simulink model "Tricopter_Controlled"  (R2012b)
settings: Solver=ode3  StartTime=0.0  StopTime=inf  FixedStep=T_sim  MaxStep=0.01  RelTol=1e-5
values from neighbouring files (symbols this model uses):
  A_l_max_x = sqrt( (Max_Thrust*3/m)^2  -  g^2  )    [Run3Copter.m]
  A_x = 0.015    [SetupComplete.m]
  A_y = A_x    (= 0.015)    [SetupComplete.m]
  A_z = 0.16    [SetupComplete.m]
  A_z_max = Max_Thrust*3/m    [Run3Copter.m]
  Alt_0 = input(' Give the initial altitude (m): ')    [Run3Copter.m]
  C_x = 1.2    [SetupComplete.m]
  C_y = C_x    (= 1.2)    [SetupComplete.m]
  C_z = 2.2    [SetupComplete.m]
  CG_0 = [0,0,0.02]'    [SetupComplete.m]
  epsilon = 0.01    [Run3Copter.m]
  eta_1 = deg2rad(-2)    [Run3Copter.m]
  eta_23 = 0    [Run3Copter.m]
  g = 9.81    [SetupComplete.m]
  h_M = 0.064    [SetupComplete.m]
  I_BAC_0 = [ Ix,0,Ixz;0,Iy,0;Ixz,0,Iz]    [SetupComplete.m]
  Initial_Omegas = Omega_hover    [Run3Copter.m]
  Initial_Torques = Torque_hover    [Run3Copter.m]
  Ix = 0.0552    [SetupComplete.m]
  Iy = 0.0552    [SetupComplete.m]
  Iz = 0.11    [SetupComplete.m]
  l = 0.345    [SetupComplete.m]
  l_arm = 0.264    [SetupComplete.m]
  latitude = 52.0733    [Run3Copter.m]
  longitude = 0.6278    [Run3Copter.m]
  m = 3.51    [SetupComplete.m]
  m_0 = 2.61    [SetupComplete.m]
  m_M = 0.300    (= 0.3)    [SetupComplete.m]
  rho = 1.15    [SetupComplete.m]
  Rotation_sign = [ 1,-1,-1]    [SetupComplete.m]
  T_sim = 0.01    [Run3Copter.m]
  throtle_1 = throtle_23/cos(eta_1)    [Run3Copter.m]
  throtle_23 = 0.745    [Run3Copter.m]
  v_i0 = sqrt( 1/3*m*g/(2*rho*pi*R^2)  )    [SetupComplete.m]
undefined symbols (not defined in the file or in its folder): DOWN_0, Earth, EAST_0, Newton, NORTH_0, P_0, Q_0, R_0, Raphson, U_0, V_0, W_0, WGS84
libraries: Adaptive_FaultTolerantControl x24, simulink_extras x11, XXCopter_C x7, XXCopter x5, aerolibfltsims x3, XXCopter_Control x2, qcatlib x1, aerolibconvert2 x1, aerolibtransform2 x1, aerolibanimutils x1, aerolibobsolete x1, simulink x1
(part 1 of 3)
settings Model: ExtModeTrigDuration=5000  Creator=DavidTorres  LastModifiedBy=david.torres
settings SolverCC: SolverResetMethod=Robust  PositivePriorityOrder=on
settings DataIOCC: ExternalInput=getinputstruct(op_trim1)  InitialState=getstatestruct(op_trim1)  SignalLoggingSaveFormat=ModelDataLogs  Refine=10
settings OptimizationCC: InlineParams=on  OptimizeModelRefInitCode=on  LifeSpan=1  SimCompilerOptimization=On
settings DebuggingCC: FcnCallInpInsideContextMsg=UseLocalSettings
settings HardwareCC: ProdIntDivRoundTo=Zero  ProdEndianess=LittleEndian  ProdHWDeviceType=Generic->32-bit x86 compatible
settings RTWCC: SystemTargetFile=ert.tlc  GenCodeOnly=on  TemplateMakefile=RTW.MSVCBuild  Description=Create Visual C/C++ Solution File for the Embedded Coder  ProcessScript=ert_make_rtw_hook
settings CodeAppCC: IgnoreCustomStorageClasses=off
settings ERTTargetCC: CodeReplacementLibrary=C89/C90 (ANSI)  MultiwordLength=2048  GenerateSampleERTMain=on  InlinedParameterPlacement=NonHierarchical  ERTCustomFileTemplate=example_file_process.tlc  ConvertIfToSwitch=off  SuppressUnreachableDefaultCases=off

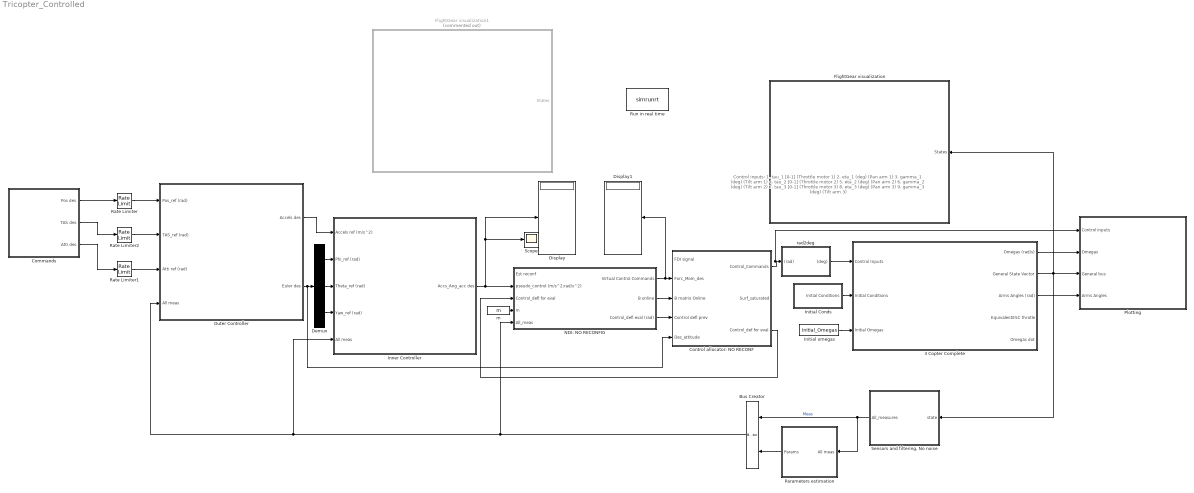
== system Tricopter_Controlled ==
  note: Control inputs:
      | 1. tau_1 [0-1] (Throttle motor 1)
      | 2. eta_1 (deg)  (Pan arm 1)
      | 3. gamma_1 (deg)  (Tilt arm 1)
      |
      | 4. tau_2 [0-1] (Throttle motor 2)
      | 5. eta_2 (deg)  (Pan arm 2)
      | 6. gamma_2 (deg)  (Tilt arm 2)
      |
      | 7. tau_3 [0-1] (Throttle motor 3)
      | 8. eta_3 (deg)  (Pan arm  3)
      | 9. gamma_3 (deg)  (Tilt arm 3)
  3 Copter Complete : Subsystem
      mask Display:
      | image(imread('conv.jpg'))
      | port_label('input', 1, 'Control_in(deg)')
      | port_label('input', 2, 'Ini_condi')
      | port_label('input', 3, 'Ini_Omegas')
      | port_label('output', 1, 'Omegas (rad/s)')
      | port_label('output', 2, 'Gen_state_vec')
      | port_label('output', 3, 'Arms_angl(rad)')
      | port_label('output', 4, 'Eq_ESC_Thro')
      | port_label('output', 5, 'Omegas_dot')
  Bus Creator : BusCreator  Inputs=2
  Commands : Subsystem  TreatAsAtomicUnit=on
  Control allocator: NO RECONF : Subsystem  RTWFcnName=abc  RTWFileName=asas  VariantObject=Control Allocator: NO RECONFIG
      settings: MinAlgLoopOccurrences=on  RTWFcnNameOpts=User specified  RTWFileNameOpts=User specified
  Demux : Demux  Outputs=3
  Display : Display
  Display1 : Display
  FlightGear visualization : Subsystem  TreatAsAtomicUnit=on
      mask Display:
      | disp('{\bf\fontsize{20} Flight Gear}', 'texmode','on');
      | image(imread('convFG.jpg'))
      | port_label('input', 1, 'States')
      | % port_label('input', 2, 'States_dot')
      | % port_label('input', 3, 'Controls')
  FlightGear visualization1 : Subsystem  Commented=on  TreatAsAtomicUnit=on
      mask Display:
      | disp('{\bf\fontsize{20} Flight Gear}', 'texmode','on');
      | image(imread('convFG.jpg'))
      | port_label('input', 1, 'States')
      | % port_label('input', 2, 'States_dot')
      | % port_label('input', 3, 'Controls')
  Initial Conds : Subsystem  TreatAsAtomicUnit=on
  Initial omegas : Constant  Value=Initial_Omegas
  Inner Controller : Subsystem  Variant=on  OverrideUsingVariant=PI
  NDI: NO RECONFIG : Subsystem  RTWFcnName=abc  RTWFileName=asas  VariantObject=NDI: NO RECONFIG
      settings: RTWFcnNameOpts=User specified  RTWFileNameOpts=User specified
  Outer Controller : Subsystem  Variant=on  OverrideUsingVariant=Overactuated P Controller
  Parameters estimation : Subsystem  TreatAsAtomicUnit=on
  Plotting : Subsystem
  Rate Limiter : RateLimiter  RisingSlewLimit=5  FallingSlewLimit=-5  SampleTimeMode=inherited
  Rate Limiter1 : RateLimiter  RisingSlewLimit=0.2  FallingSlewLimit=-0.2  SampleTimeMode=inherited
  Rate Limiter2 : RateLimiter  RisingSlewLimit=10  FallingSlewLimit=-10  SampleTimeMode=inherited
  Run in real time : S-Function  FunctionName=simrunrt  Parameters=1  EnableBusSupport=off
  Scope : Scope
      settings: YMin=-2  YMax=8  SaveName=ScopeData3
  Sensors and filtering. No noise : Subsystem  VariantObject=No noise
  m : Constant  Value=m
  rad2deg : Subsystem  TreatAsAtomicUnit=on
  wires:
  Initial omegas/1 -> 3 Copter Complete/3(Initial Omegas)
  Initial Conds/1(Initial Conditions) -> 3 Copter Complete/2(Initial Conditions)
  3 Copter Complete/2(General State Vector) -> Sensors and filtering. No noise/1(state), Plotting/3(General bus), FlightGear visualization/1(States)
  3 Copter Complete/1(Omegas (rad/s)) -> Plotting/2(Omegas)
  Control allocator: NO RECONF/1(Control_Commands) -> Plotting/1(Control inputs), rad2deg/1((rad))
  NDI: NO RECONFIG/1(Virtual Control Commands) -> Display1/1, Control allocator: NO RECONF/2(Forc_Mom_des)
  Control allocator: NO RECONF/3(Control_def for eval) -> NDI: NO RECONFIG/3(Control_defl for eval)
  m/1 -> NDI: NO RECONFIG/4(m)
  NDI: NO RECONFIG/3(Control_defl eval (rad)) -> Control allocator: NO RECONF/4(Control defl prev)
  rad2deg/1((deg)) -> 3 Copter Complete/1(Control Inputs)
  Sensors and filtering. No noise/1(All_measures) -> Parameters estimation/1(All meas), Bus Creator/1  "Meas"
  NDI: NO RECONFIG/2(B online) -> Control allocator: NO RECONF/3(B matrix Online)
  Inner Controller/1(Accs_Ang_acc des) -> Display/1, Scope/1, NDI: NO RECONFIG/2(pseudo_control (m/s^2;rad/s^2))
  Parameters estimation/1(Params) -> Bus Creator/2
  3 Copter Complete/3(Arms Angles (rad)) -> Plotting/4(Arms Angles)
  Bus Creator/1 -> Outer Controller/4(All meas), Inner Controller/5(All meas), NDI: NO RECONFIG/5(All_meas)
  Outer Controller/2(Euler des) -> Control allocator: NO RECONF/5(Des_attitude), Demux/1
  Demux/3 -> Inner Controller/4(Yaw_ref (rad))
  Demux/2 -> Inner Controller/3(Theta_ref (rad))
  Demux/1 -> Inner Controller/2(Phi_ref (rad))
  Outer Controller/1(Accels des) -> Inner Controller/1(Accels ref (m/s^2))
  Commands/1(Pos des) -> Rate Limiter/1
  Rate Limiter/1 -> Outer Controller/1(Pos_ref (rad))
  Commands/3(Atti des) -> Rate Limiter1/1
  Rate Limiter1/1 -> Outer Controller/3(Atti ref (rad))
  Rate Limiter2/1 -> Outer Controller/2(TAS_ref (rad))
  Commands/2(TAS des) -> Rate Limiter2/1

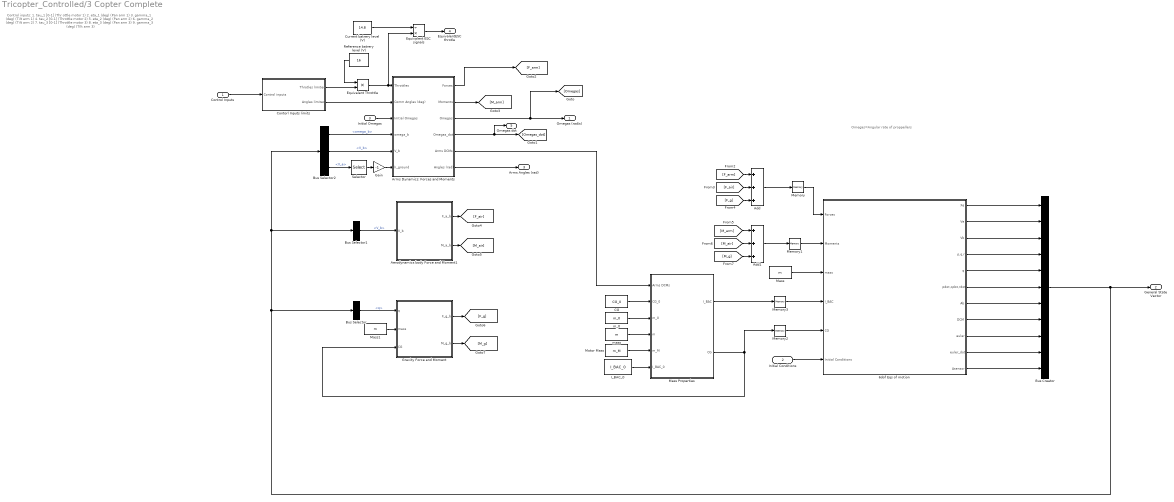
== system Tricopter_Controlled/3 Copter Complete ==
  note: Omegas=Angular rate of proppellers
  note: Control inputs:
      | 1. tau_1 [0-1] (Thr ottle motor 1)
      | 2. eta_1 (deg)  (Pan arm 1)
      | 3. gamma_1 (deg)  (Tilt arm 1)
      |
      | 4. tau_2 [0-1] (Throttle motor 2)
      | 5. eta_2 (deg)  (Pan arm 2)
      | 6. gamma_2 (deg)  (Tilt arm 2)
      |
      | 7. tau_3 [0-1] (Throttle motor 3)
      | 8. eta_3 (deg)  (Pan arm  3)
      | 9. gamma_3 (deg)  (Tilt arm 3)
  Control Inputs : Inport
  Initial Conditions : Inport  Port=2
  Initial Omegas : Inport  Port=3
  6dof Eqs of motion : Subsystem  TreatAsAtomicUnit=on
  Add : Sum  Inputs=+++
  Add1 : Sum  Inputs=+++
  Aerodynamics body Force and Moment1 : MATLAB Function  TreatAsAtomicUnit=on
      settings: PermitHierarchicalResolution=ParametersOnly
  Arms Dynamics: Forces and Moments : Subsystem
  Bus Creator : BusCreator  Inputs=11
  Bus Selector : BusSelector  OutputSignals=q
  Bus Selector1 : BusSelector  OutputSignals=V_b
  Bus Selector2 : BusSelector  OutputSignals=omega_b,V_b,X_e
  CG : Constant  Value=CG_0
  Contorl Inputs limits : Subsystem  TreatAsAtomicUnit=on
  Current batrery level (V) : Constant  Value=14.8
  Equivalent ESC signals : Product  Inputs=/*
  Equivalent Throttle : Product  Inputs=**
  Gain : Gain  Gain=-1
  Gravity Force and Moment : MATLAB Function  TreatAsAtomicUnit=on
      settings: PermitHierarchicalResolution=ParametersOnly
  I_BAC_0 : Constant  Value=I_BAC_0
  Mass : Constant  Value=m
  Mass Properties : Subsystem  TreatAsAtomicUnit=on
  Mass1 : Constant  Value=m
  Memory : Memory  X0=[0,0,0]
  Memory1 : Memory  X0=[0,0,0]
  Memory2 : Memory  X0=CG_0
  Memory3 : Memory  X0=I_BAC_0
  Motor Mass : Constant  Value=m_M
  Reference batrery level (V) : Constant  Value=16
  Selector : Selector  InputPortWidth=3  Indices=3
  m_0 : Constant  Value=m_0
  mass : Constant  Value=m
  Omegas (rad/s) : Outport
  General State Vector : Outport  Port=2
  Arms Angles (rad) : Outport  Port=3
  EquivalentESC throtle : Outport  Port=4
  Omegas dot : Outport  Port=5
  wires:
  Initial Conditions/1 -> 6dof Eqs of motion/6(Initial Conditions)
  6dof Eqs of motion/3(Vb) -> Bus Creator/3
  6dof Eqs of motion/5(q) -> Bus Creator/5
  6dof Eqs of motion/2(Ve) -> Bus Creator/2
  6dof Eqs of motion/6(pdot,qdot,rdot) -> Bus Creator/6
  6dof Eqs of motion/1(Xe) -> Bus Creator/1
  6dof Eqs of motion/7(Ab) -> Bus Creator/7
  6dof Eqs of motion/8(DCM) -> Bus Creator/8
  6dof Eqs of motion/9(euler) -> Bus Creator/9
  6dof Eqs of motion/10(euler_dot) -> Bus Creator/10
  Bus Selector/1 -> Gravity Force and Moment/1(q)  "<q>"
  Mass/1 -> 6dof Eqs of motion/3(mass)
  Mass Properties/1(I_BAC) -> Memory3/1
  Bus Selector1/1 -> Aerodynamics body Force and Moment1/1(V_b)  "<V_b>"
  Bus Selector2/1 -> Arms Dynamics: Forces and Moments/4(omega_b)  "<omega_b>"
  Bus Selector2/2 -> Arms Dynamics: Forces and Moments/5(V_b)  "<V_b>"
  Mass1/1 -> Gravity Force and Moment/2(mass)
  Mass Properties/2(CG) -> Gravity Force and Moment/3(CG), Memory2/1
  Arms Dynamics: Forces and Moments/4(Omegas_dot) -> Omegas dot/1, [Omegas_dot]
  Initial Omegas/1 -> Arms Dynamics: Forces and Moments/3(Initial Omegas)
  Bus Selector2/3 -> Selector/1  "<X_e>"
  Selector/1 -> Gain/1
  Gain/1 -> Arms Dynamics: Forces and Moments/6(h_ground)
  Add/1 -> Memory/1
  Add1/1 -> Memory1/1
  Arms Dynamics: Forces and Moments/1(Forces) -> [F_arm]
  Arms Dynamics: Forces and Moments/2(Moments) -> [M_arm]
  Aerodynamics body Force and Moment1/1(F_a_b) -> [F_air]
  Aerodynamics body Force and Moment1/2(M_a_b) -> [M_air]
  Gravity Force and Moment/1(F_g_b) -> [F_g]
  Gravity Force and Moment/2(M_g_b) -> [M_g]
  [F_arm] -> Add/1
  [F_air] -> Add/2
  [F_g] -> Add/3
  [M_arm] -> Add1/1
  [M_g] -> Add1/3
  [M_air] -> Add1/2
  6dof Eqs of motion/11(Asensor) -> Bus Creator/11
  Contorl Inputs limits/1(Throtles limited) -> Equivalent Throttle/2
  Contorl Inputs limits/2(Angles limited) -> Arms Dynamics: Forces and Moments/2(Comm Angles (deg))
  Arms Dynamics: Forces and Moments/5(Arms DCMs) -> Mass Properties/1(Arms DCMs)
  CG/1 -> Mass Properties/2(CG_0)
  Motor Mass/1 -> Mass Properties/5(m_M)
  I_BAC_0/1 -> Mass Properties/6(I_BAC_0)
  m_0/1 -> Mass Properties/3(m_0)
  mass/1 -> Mass Properties/4(m)
  Arms Dynamics: Forces and Moments/3(Omegas) -> [Omegas], Omegas (rad/s)/1
  Bus Creator/1 -> Bus Selector2/1, Bus Selector1/1, Bus Selector/1, General State Vector/1
  Memory/1 -> 6dof Eqs of motion/1(Forces)
  Memory1/1 -> 6dof Eqs of motion/2(Moments)
  Memory2/1 -> 6dof Eqs of motion/5(CG)
  Memory3/1 -> 6dof Eqs of motion/4(I_BAC)
  Equivalent Throttle/1 -> Equivalent ESC signals/2, Arms Dynamics: Forces and Moments/1(Throttles)
  Reference batrery level (V)/1 -> Equivalent Throttle/1
  Current batrery level (V)/1 -> Equivalent ESC signals/1
  Equivalent ESC signals/1 -> EquivalentESC throtle/1
  6dof Eqs of motion/4(p,q,r) -> Bus Creator/4
  Arms Dynamics: Forces and Moments/6(Angles (rad)) -> Arms Angles (rad)/1
  Control Inputs/1 -> Contorl Inputs limits/1(Control inputs)

== system Tricopter_Controlled/Commands ==
  Ini Position X_e_0 : Constant  Value=[0;0;-Alt_0-10]
  Ini Position X_e_1 : Constant  Value=[0;0;-Alt_0]
  Initial Attitude Euler_0 : Constant  Value=[deg2rad(0);deg2rad(0);deg2rad(90)]  SampleTime=-1
  Initial Attitude Euler_1 : Constant  Value=[deg2rad(0);deg2rad(0);deg2rad(0)]
  Manual Switch : ManualSwitch  CurrentSetting=0
  Manual Switch1 : ManualSwitch
  Manual Switch2 : ManualSwitch  CurrentSetting=0
  Veas des : Constant  Value=0
  Veas des1 : Constant  Value=10
  Pos des : Outport
  TAS des : Outport  Port=2
  Atti des : Outport  Port=3
  wires:
  Manual Switch1/1 -> Pos des/1
  Manual Switch/1 -> Atti des/1
  Initial Attitude Euler_0/1 -> Manual Switch/1
  Initial Attitude Euler_1/1 -> Manual Switch/2
  Ini Position X_e_0/1 -> Manual Switch1/1
  Ini Position X_e_1/1 -> Manual Switch1/2
  Manual Switch2/1 -> TAS des/1
  Veas des1/1 -> Manual Switch2/1
  Veas des/1 -> Manual Switch2/2

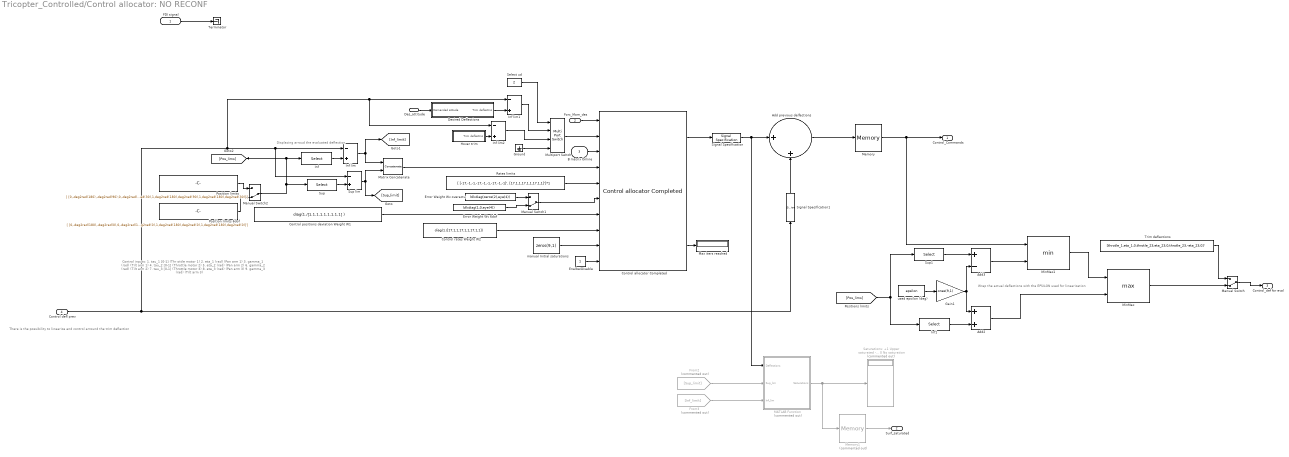
== system Tricopter_Controlled/Control allocator: NO RECONF ==
  note: There is the possibility to linearize and control arround the trim deflection
  note: Wrap the actual deflections with the EPSILON
      |  used for linearization
  note: Displacing arroud the evaluated deflection
  note: Control inputs:
      | 1. tau_1 [0-1] (Thr ottle motor 1)
      | 2. eta_1 (rad)  (Pan arm 1)
      | 3. gamma_1 (rad)  (Tilt arm 1)
      |
      | 4. tau_2 [0-1] (Throttle motor 2)
      | 5. eta_2 (rad)  (Pan arm 2)
      | 6. gamma_2 (rad)  (Tilt arm 2)
      |
      | 7. tau_3 [0-1] (Throttle motor 3)
      | 8. eta_3 (rad)  (Pan arm  3)
      | 9. gamma_3 (rad)  (Tilt arm 3)
  FDI signal : Inport
  Forc_Mom_des : Inport  Port=2
  B matrix Online : Inport  Port=3
  Control defl prev : Inport  Port=4
  Des_attitude : Inport  Port=5
  Add previous delfections : Sum  Inputs=|++
  Add2 : Sum
  Add3 : Sum  Inputs=+-
  "Control allocator Completed " : qcatlib/Control allocator Completed   alg=WLS  CA_type=QP  iter_max=100  gamma=1  k_B=6  m_B=9  T=T_sim  tol=1e-5
  Control positions deviation Weight W1 : Constant  Value=diag(1./[1,1,1,1,1,1,1,1,1] )
  Control rates Weight W2 : Constant  Value=diag(1./[17,1,1,17,1,1,17,1,1])
  Desired Deflections : Subsystem  TreatAsAtomicUnit=on
  Enalbe/Disable : Constant
  Error Weight Wv 6dof : Constant  Value=blkdiag(1,0,eye(4))
  Error Weight Wv overactu : Constant  Value=blkdiag(zeros(2),eye(4))
  From2 : From  Commented=on  GotoTag=Sup_limit
  From3 : From  Commented=on  GotoTag=Inf_limit
  Gain1 : Gain  Gain=ones(9,1)
  Ground : Ground
  Hover trim : Subsystem  TreatAsAtomicUnit=on
  Inf : Selector  NumberOfDimensions=2  InputPortWidth=3  IndexOptions=Index vector (dialog),Index vector (dialog)  Indices=[1:9],1  OutputSizes=1,1
  Inf lim : Sum  Inputs=-+
  Inf lim1 : Sum  Inputs=-+
  Inf lim2 : Sum  Inputs=-+
  Inf1 : Selector  NumberOfDimensions=2  InputPortWidth=3  IndexOptions=Index vector (dialog),Index vector (dialog)  Indices=[1:9],1  OutputSizes=1,1
  MATLAB Function : MATLAB Function  Commented=on  TreatAsAtomicUnit=on
      settings: PermitHierarchicalResolution=ParametersOnly
  Manual Switch : ManualSwitch  CurrentSetting=0
  Manual Switch1 : ManualSwitch  CurrentSetting=0
  Manual Switch2 : ManualSwitch  CurrentSetting=0
  Matrix Concatenate : Concatenate  Mode=Multidimensional array  ConcatenateDimension=2
  Max iters reached : Display
  Memory : Memory  X0=[throtle_1,eta_1,0,throtle_23,eta_23,0,throtle_23,-eta_23,0]'
  Memory1 : Memory  Commented=on  X0=zeros(7,1)
  MinMax : MinMax  Function=max  Inputs=2
  MinMax1 : MinMax  Inputs=2
  Multiport Switch : MultiPortSwitch
  Position limits : Constant  Value=[ [0,-deg2rad(180),-deg2rad(90),0,-deg2rad(180),-deg2rad(30),0,-deg2rad(180),-deg2rad(90)]', [1,deg2rad(180),deg2rad(30),1,deg2rad(180),deg2rad(90),1,deg2rad(180),deg2rad(30)]']
  Position limits 6dof : Constant  Value=[ [0,-deg2rad(180),-deg2rad(0),0,-deg2rad(180),-deg2rad(0),0,-deg2rad(180),-deg2rad(0)]', [1,deg2rad(180),deg2rad(0),1,deg2rad(180),deg2rad(0),1,deg2rad(180),deg2rad(0)]']
  Rates limits : Constant  Value=[ [-17,-1,-1,-17,-1,-1,-17,-1,-1]', [17,1,1,17,1,1,17,1,1]']*1
  Saturations: +1 Upper saturated -1 Lower saturated 0 No saturation : Display  Commented=on
  Select ud : Constant  Value=2
  Signal Specification : SignalSpecification  Dimensions=[9,1]
  Signal Specification1 : SignalSpecification  Dimensions=[9,1]
  Sup : Selector  NumberOfDimensions=2  InputPortWidth=3  IndexOptions=Index vector (dialog),Index vector (dialog)  Indices=[1:9],2  OutputSizes=1,1
  Sup lim : Sum  Inputs=-+
  Sup1 : Selector  NumberOfDimensions=2  InputPortWidth=3  IndexOptions=Index vector (dialog),Index vector (dialog)  Indices=[1:9],2  OutputSizes=1,1
  Terminator : Terminator
  "Trim deflections " : Constant  Value=[throtle_1,eta_1,0,throtle_23,eta_23,0,throtle_23,-eta_23,0]'
  manual Initial saturations : Constant  Value=zeros(9,1)
  used epsilon (deg) : Constant  Value=epsilon
  Control_Commands : Outport
  Surf_saturated : Outport  Port=2
  Control_def for eval : Outport  Port=3
  wires:
  Manual Switch/1 -> Control_def for eval/1
  MinMax1/1 -> MinMax/1
  Add3/1 -> MinMax1/2
  used epsilon (deg)/1 -> Gain1/1
  Inf1/1 -> Add2/2
  Gain1/1 -> Add3/2, Add2/1
  Sup1/1 -> Add3/1
  Add2/1 -> MinMax/2
  Add previous delfections/1 -> Memory/1
  Control positions deviation Weight W1/1 -> "Control allocator Completed "/7
  FDI signal/1 -> Terminator/1
  "Control allocator Completed "/1 -> Signal Specification/1
  Enalbe/Disable/1 -> "Control allocator Completed "/10
  manual Initial saturations/1 -> "Control allocator Completed "/9
  "Control allocator Completed "/3 -> Max iters reached/1
  Sup lim/1 -> [Sup_limit], Matrix Concatenate/2
  Inf lim/1 -> [Inf_limit], Matrix Concatenate/1
  Inf/1 -> Inf lim/2
  Sup/1 -> Sup lim/2
  Control rates Weight W2/1 -> "Control allocator Completed "/8
  Manual Switch1/1 -> "Control allocator Completed "/6
  Rates limits/1 -> "Control allocator Completed "/5
  Manual Switch2/1 -> Inf/1, [Pos_lims], Sup/1
  Memory/1 -> MinMax1/1, Control_Commands/1
  From2/1 -> MATLAB Function/2(Sup_lim)
  From3/1 -> MATLAB Function/3(Inf_lim)
  MATLAB Function/1(Saturations) -> Memory1/1, Saturations: +1 Upper saturated -1 Lower saturated 0 No saturation/1
  Memory1/1 -> Surf_saturated/1
  B matrix Online/1 -> "Control allocator Completed "/3
  Signal Specification/1 -> MATLAB Function/1(Deflections), Add previous delfections/1
  Signal Specification1/1 -> Add previous delfections/2
  Desired Deflections/1(Trim deflectins) -> Inf lim1/2
  [Pos_lims] -> Sup1/1, Inf1/1
  Forc_Mom_des/1 -> "Control allocator Completed "/1
  "Trim deflections "/1 -> Manual Switch/1
  MinMax/1 -> Manual Switch/2
  Matrix Concatenate/1 -> "Control allocator Completed "/4
  Multiport Switch/1 -> "Control allocator Completed "/2
  Error Weight Wv overactu/1 -> Manual Switch1/1
  Des_attitude/1 -> Desired Deflections/1(Demanded atitude)
  Hover trim/1(Trim deflectins) -> Inf lim2/2
  Control defl prev/1 -> Signal Specification1/1, Inf lim2/1, Inf lim1/1, Inf lim/1, Sup lim/1
  Inf lim1/1 -> Multiport Switch/2
  Inf lim2/1 -> Multiport Switch/3
  Ground/1 -> Multiport Switch/4
  Select ud/1 -> Multiport Switch/1
  Position limits 6dof/1 -> Manual Switch2/2
  Position limits/1 -> Manual Switch2/1
  Error Weight Wv 6dof/1 -> Manual Switch1/2

== system Tricopter_Controlled/FlightGear visualization ==
  States : Inport
  Bus Selector : BusSelector  OutputSignals=X_e,euler
  Demux : Demux  Outputs=3
  Flat Earth to LLA : Subsystem
  Mux : Mux  Inputs=6
  Saturation : Saturate  UpperLimit=1e8  LowerLimit=-1e5  OutDataTypeStr=double
  Send2FG : S-Function  FunctionName=sim2fg  Parameters='localhost',5502  EnableBusSupport=off
  cast1 : DataTypeConversion  OutDataTypeStr=double  SaturateOnIntegerOverflow=on
  href : Constant  Value=Alt_0  VectorParams1D=off
  keep pi/pi : Subsystem
  wires:
  States/1 -> Bus Selector/1
  Demux/2 -> Mux/5
  Demux/1 -> Mux/4
  href/1 -> Flat Earth to LLA/2(altitude0)
  Saturation/1 -> Mux/3
  Mux/1 -> cast1/1
  cast1/1 -> Send2FG/1
  keep pi/pi/1(ptp_earth) -> Demux/1
  Demux/3 -> Mux/6
  Flat Earth to LLA/3(altitude h) -> Saturation/1
  Flat Earth to LLA/1(latitude mu) -> Mux/1
  Flat Earth to LLA/2(longitude l) -> Mux/2
  Bus Selector/2 -> keep pi/pi/1(phi theta psi)  "<euler>"
  Bus Selector/1 -> Flat Earth to LLA/1(Xe)  "<X_e>"

== system Tricopter_Controlled/FlightGear visualization1 ==
  States : Inport
  Bus Selector : BusSelector  OutputSignals=X_e,omega_b,euler
  Demux : Demux  Outputs=3
  Flat Earth to LLA : Subsystem
  Generate Run Script (Cranfield Airport) : aerolibfltsims/Generate Run Script  OutputFileName=runfg.bat  FlightGearBaseDirectory=C:\Program Files\FlightGear  GeometryModelName=f16  DestinationPort=5502  OriginAddress=127.0.0.1  OriginPort=5505  LocalAddress=127.0.0.1  AirportId=EGTC  RunwayId=1  InitialAltitude=Alt_0*3.2808399  InitialHeading=0  OffsetDistance=1  OffsetAzimuth=0  GenerateFile=off  Architecture=Win64  dataFlow=Send
  Pack net_fdm Packet for FlightGear : aerolibfltsims/Pack net_fdm Packet for FlightGear  FlightGearVersion=v2.6  ShowPositionAttitudeInputs=on  ShowVelocityAccelerationInputs=off  ShowControlSurfacePositionInputs=off  ShowEngineFuelInputs=off  ShowLandingGearInputs=off  ShowEnvironmentInputs=off  SampleTime=-1
      settings: AttributesFormatString=FG VERSION: %<FlightGearVersion>
  Saturation : Saturate  UpperLimit=1e8  LowerLimit=-1e5
  Send net_fdm Packet to FlightGear : aerolibfltsims/Send net_fdm Packet to FlightGear  DestinationIpAddress=127.0.0.1  DestinationPort=5502  LocalIpPort=-1  varLen=off  SampleTime=-1
  Simulation Pace : aerolibanimutils/Simulation Pace  SimulationPace=1  SleepMode=MATLAB Thread  OutputPaceError=off  SampleTime=4*T_sim
      settings: AttributesFormatString=%<SimulationPace> sec/sec
  cast2 : DataTypeConversion  OutDataTypeStr=single  SaturateOnIntegerOverflow=on
  href : Constant  Value=Alt_0  VectorParams1D=off
  phidot thetadot psidot : Subsystem
  wires:
  Bus Selector/3 -> phidot thetadot psidot/2(phi theta psi)  "<euler>"
  Bus Selector/2 -> phidot thetadot psidot/1(pqr)  "<omega_b>"
  Bus Selector/1 -> Flat Earth to LLA/1(Xe)  "<X_e>"
  States/1 -> Bus Selector/1
  Demux/3 -> Pack net_fdm Packet for FlightGear/6
  Demux/2 -> Pack net_fdm Packet for FlightGear/5
  Demux/1 -> Pack net_fdm Packet for FlightGear/4
  Saturation/1 -> Pack net_fdm Packet for FlightGear/3
  cast2/1 -> Demux/1
  Flat Earth to LLA/2(latitude mu) -> Pack net_fdm Packet for FlightGear/2
  Flat Earth to LLA/1(longitude l) -> Pack net_fdm Packet for FlightGear/1
  Flat Earth to LLA/3(altitude h) -> Saturation/1
  href/1 -> Flat Earth to LLA/2(altitude0)
  phidot thetadot psidot/1(ptp_earth) -> cast2/1
  Pack net_fdm Packet for FlightGear/1 -> Send net_fdm Packet to FlightGear/1

== system Tricopter_Controlled/Initial Conds ==
  Bus Creator : BusCreator
  Ini Position X_e_0 : Constant  Value=[0;0;-Alt_0]
  Initial Attitude Euler_0 : Constant  Value=[deg2rad(0);deg2rad(0);deg2rad(0)]
  Initial Attitude Rate  Euler_dot_0 : Constant  Value=[deg2rad(0);deg2rad(0);deg2rad(0)]
  Initial Velocity V_e_0 : Constant  Value=[0;0;0]
  Initial Conditions : Outport
  wires:
  Ini Position X_e_0/1 -> Bus Creator/1  "X_e_0"
  Initial Velocity V_e_0/1 -> Bus Creator/2  "V_e_0"
  Initial Attitude Euler_0/1 -> Bus Creator/3  "Euler_0"
  Initial Attitude Rate  Euler_dot_0/1 -> Bus Creator/4  "Euler_dot_0"
  Bus Creator/1 -> Initial Conditions/1

== system Tricopter_Controlled/Inner Controller ==
  note: 1) Only subsystems can be added as variant choices at this level
      | 2) Blocks cannot be connected at this level as connectivity is
      | automatically determined at simulation, based on the active variant
  Accels ref (m/s^2) : Inport
  Phi_ref (rad) : Inport  Port=2
  Theta_ref (rad) : Inport  Port=3
  Yaw_ref (rad) : Inport  Port=4
  All meas : Inport  Port=5
  P Controller : Subsystem  VariantObject=P
  PI Controller : Subsystem  VariantObject=PI
  Accs_Ang_acc des : Outport

== system Tricopter_Controlled/NDI: NO RECONFIG ==
  note: Rejection for the
      | angular accelerations
  note: Pseudo control inputs:
      | 1. Desired angular accelerations (rad/s^2)
      | 2. Desired accelerations (m/s^2) in body axes
  Est reconf : Inport
  pseudo_control (m/s^2;rad/s^2) : Inport  Port=2
  Control_defl for eval : Inport  Port=3
  m : Inport  Port=4
  All_meas : Inport  Port=5
  3Copter_4_NDI&CA : Subsystem  AncestorBlock=XXCopter_Control/3Copter_4_NDI&CA  TreatAsAtomicUnit=on
  Bus Selector : BusSelector  OutputSignals=Meas.omega_b meas (rad/s),Meas.q_meas,Meas.V_b_meas,Meas.Alt meas (m)
  Demux : Demux  Outputs=[3,3]
  Derivative1 : Derivative  CoefficientInTFapproximation=500
  Gain : Gain  Gain=[1,0,1]
  Gain1 : Gain  Gain=[1,0,1]'
  Ground : Ground
  Ground1 : Ground
  Inversion : Sum  Inputs=|+-
  Mux : Mux  Inputs=[3,3]
  Mux2 : Mux  Inputs=[3,3]
  Rot eqs_ Get moments : XXCopter_Control/Rot eqs_ Get moments
  Terminator : Terminator
  Transl Eqs_ Get forces : XXCopter_Control/Transl Eqs_ Get forces
  "angles " : Selector  IndexMode=Zero-based  InputPortWidth=9  Indices=[1,2,4,5,7,8]
  epsilon (rad or unitary) : Constant  Value=epsilon
  m1 : InportShadow  Port=4
  Virtual Control Commands : Outport
  B online : Outport  Port=2
  Control_defl eval (rad) : Outport  Port=3
  wires:
  Est reconf/1 -> Terminator/1
  3Copter_4_NDI&CA/3(CA_grad) -> B online/1
  Mux/1 -> Inversion/1
  Mux2/1 -> Inversion/2  "f_x(x)"
  All_meas/1 -> Bus Selector/1
  pseudo_control (m/s^2;rad/s^2)/1 -> Demux/1
  Demux/2 -> Rot eqs_ Get moments/2, Transl Eqs_ Get forces/4
  Demux/1 -> Transl Eqs_ Get forces/1
  Bus Selector/1 -> Transl Eqs_ Get forces/3, Rot eqs_ Get moments/1, 3Copter_4_NDI&CA/6(omega_b)  "<omega_b meas (rad/s)>"
  Bus Selector/3 -> Transl Eqs_ Get forces/2, 3Copter_4_NDI&CA/4(Vb)  "<V_b_meas>"
  3Copter_4_NDI&CA/4(I_BAC) -> Rot eqs_ Get moments/3
  3Copter_4_NDI&CA/5("CG ") -> Transl Eqs_ Get forces/6
  Control_defl for eval/1 -> 3Copter_4_NDI&CA/2(Control Inputs (rad)), Control_defl eval (rad)/1, "angles "/1
  Bus Selector/4 -> 3Copter_4_NDI&CA/3(h)  "<Alt meas (m)>"
  Bus Selector/2 -> 3Copter_4_NDI&CA/5(q)  "<q_meas>"
  m/1 -> 3Copter_4_NDI&CA/11(" m")
  m1/1 -> Transl Eqs_ Get forces/5
  epsilon (rad or unitary)/1 -> 3Copter_4_NDI&CA/1("epsilon (rad or unitary) ")
  Transl Eqs_ Get forces/1 -> Gain1/1
  Rot eqs_ Get moments/1 -> Mux/2
  3Copter_4_NDI&CA/1(Forces) -> Gain/1
  3Copter_4_NDI&CA/2(Moments) -> Mux2/2
  Inversion/1 -> Virtual Control Commands/1
  Ground/1 -> 3Copter_4_NDI&CA/7(Omegas_dot_actual)
  "angles "/1 -> Derivative1/1, 3Copter_4_NDI&CA/8(angles_actual)
  Derivative1/1 -> 3Copter_4_NDI&CA/9(angles_dot_actual)
  Ground1/1 -> 3Copter_4_NDI&CA/10(angles_dot_dot_actual)
  Gain/1 -> Mux2/1
  Gain1/1 -> Mux/1

== system Tricopter_Controlled/Outer Controller ==
  note: 1) Only subsystems can be added as variant choices at this level
      | 2) Blocks cannot be connected at this level as connectivity is
      | automatically determined at simulation, based on the active variant
  Pos_ref (rad) : Inport
  TAS_ref (rad) : Inport  Port=2
  Atti ref (rad) : Inport  Port=3
  All meas : Inport  Port=4
  Overactuated P Controller : Subsystem  VariantObject=Overactuated P Controller
  Underactuated P Controller : Subsystem  VariantObject=Underactuated P Controller
  Accels des : Outport
  Euler des : Outport  Port=2

== system Tricopter_Controlled/Parameters estimation ==
  All meas : Inport
  Bus Selector : BusSelector  OutputSignals=Euler meas (rad)
  DCM1 : Subsystem  TreatAsAtomicUnit=on
  Selector7 : Selector  InputPortWidth=3  Indices=[3 2 1]
  Params : Outport
  wires:
  All meas/1 -> Bus Selector/1
  Bus Selector/1 -> Selector7/1  "<Euler meas (rad)>"
  DCM1/1(DCM) -> Params/1  "DCM"
  Selector7/1 -> DCM1/1(Euler)

== system Tricopter_Controlled/Plotting ==
  Control inputs : Inport
  Omegas : Inport  Port=2
  General bus : Inport  Port=3
  Arms Angles : Inport  Port=4
  Actual ang arm 1 : simulink_extras/Transformations/Radians to Degrees
  Actual ang arm2 : simulink_extras/Transformations/Radians to Degrees
  Actual ang arm3 : simulink_extras/Transformations/Radians to Degrees
  Arms dynamics : Scope  NumInputPorts=3
      settings: ShowLegends=on  TimeRange=50  YMin=-2.5~-6.5~-6.5  YMax=0~1~1.5  SaveName=ScopeData2
  Bus Selector : BusSelector  OutputSignals=euler,omega_b,X_e,V_e,DCM
  Bus Selector1 : BusSelector  OutputSignals=Angles Arm 1,Angles Arm 2,Angles Arm 3
  Comm ang arm1 : simulink_extras/Transformations/Radians to Degrees
  Comm ang arm2 : simulink_extras/Transformations/Radians to Degrees
  Comm ang arm3 : simulink_extras/Transformations/Radians to Degrees
  Demux : Demux  Outputs=3
  Euler omega_b : Scope  NumInputPorts=2
      settings: ShowLegends=on  TimeRange=50  YMin=-5~-0.1  YMax=10~0.1
  Mux : Mux  Inputs=3
  Mux1 : Mux  Inputs=2
  Mux2 : Mux  Inputs=2
  Mux3 : Mux  Inputs=2
  Position Velocity : Scope  NumInputPorts=2
      settings: ShowLegends=on  TimeRange=50  YMin=-200~-5  YMax=100~10  SaveName=ScopeData8
  Radians to Degrees : simulink_extras/Transformations/Radians to Degrees
  Rotors states : Scope  NumInputPorts=2
      settings: ShowLegends=on  TimeRange=50  YMin=0.4~500  YMax=1~800
  angles arm 2 : Selector  InputPortWidth=9  Indices=[5,6]
  angles arm 3 : Selector  InputPortWidth=9  Indices=[8,9]
  "angles arm2 " : Selector  InputPortWidth=9  Indices=[2,3]
  throtles : Selector  InputPortWidth=9  Indices=[1,4,7]
  wires:
  General bus/1 -> Bus Selector/1
  Bus Selector/1 -> Radians to Degrees/1  "<euler>"
  Omegas/1 -> Rotors states/2  "Omegas"
  Arms Angles/1 -> Bus Selector1/1
  Mux3/1 -> Arms dynamics/3
  Mux2/1 -> Arms dynamics/2
  Mux1/1 -> Arms dynamics/1
  Bus Selector/3 -> Position Velocity/1  "<X_e>"
  Demux/3 -> Mux/3  "psi(deg)"
  Demux/1 -> Mux/1  "phi(deg)"
  Demux/2 -> Mux/2  "theta(deg)"
  Mux/1 -> Euler omega_b/1
  Bus Selector/2 -> Euler omega_b/2  "<omega_b>"
  Control inputs/1 -> "angles arm2 "/1, angles arm 3/1, angles arm 2/1, throtles/1
  Bus Selector1/1 -> Actual ang arm 1/1  "<Angles Arm 1>"
  "angles arm2 "/1 -> Comm ang arm1/1
  Bus Selector1/2 -> Actual ang arm2/1  "<Angles Arm 2>"
  angles arm 2/1 -> Comm ang arm2/1
  Bus Selector1/3 -> Actual ang arm3/1  "<Angles Arm 3>"
  angles arm 3/1 -> Comm ang arm3/1
  throtles/1 -> Rotors states/1
  Radians to Degrees/1 -> Demux/1
  Comm ang arm1/1 -> Mux1/2
  Actual ang arm3/1 -> Mux3/1
  Actual ang arm2/1 -> Mux2/1
  Actual ang arm 1/1 -> Mux1/1
  Comm ang arm2/1 -> Mux2/2
  Comm ang arm3/1 -> Mux3/2
  Bus Selector/4 -> Position Velocity/2  "<V_e>"

== system Tricopter_Controlled/Sensors and filtering. No noise ==
  state : Inport
  Bus Creator : BusCreator  Inputs=8
  Bus Selector2 : BusSelector  OutputSignals=X_e,V_b,V_e,omega_b,q,euler,A_s
  Demux : Demux  Outputs=3
  Gain{1..7} (7 alike) : Gain
  Gain8 : Gain  Gain=-1
  Terminator : Terminator
  Terminator1 : Terminator
  All_measures : Outport
  wires:
  state/1 -> Bus Selector2/1
  Bus Selector2/1 -> Gain6/1, Demux/1  "<X_e>"
  Gain8/1 -> Bus Creator/2  "Alt meas (m)"
  Demux/1 -> Terminator/1
  Demux/2 -> Terminator1/1
  Bus Selector2/2 -> Gain7/1  "<V_b>"
  Bus Selector2/4 -> Gain3/1  "<omega_b>"
  Bus Selector2/6 -> Gain2/1  "<euler>"
  Gain7/1 -> Bus Creator/3  "V_b_meas"
  Gain3/1 -> Bus Creator/5  "omega_b meas (rad/s)"
  Bus Creator/1 -> All_measures/1
  Demux/3 -> Gain8/1  "Alt meas (m)"
  Gain2/1 -> Bus Creator/7  "Euler meas (rad)"
  Bus Selector2/7 -> Gain1/1  "<A_s>"
  Gain1/1 -> Bus Creator/8  "A_accel meas"
  Bus Selector2/3 -> Gain4/1  "<V_e>"
  Gain4/1 -> Bus Creator/4  "V_e_meas"
  Bus Selector2/5 -> Gain5/1  "<q>"
  Gain5/1 -> Bus Creator/6  "q_meas"
  Gain6/1 -> Bus Creator/1  "Pos meas (m)"

== system Tricopter_Controlled/rad2deg ==
  (rad) : Inport
  Demux : Demux  Outputs=6
  Demux1 : Demux  Outputs=3
  Mux : Mux  Inputs=9
  Radians to Degrees : simulink_extras/Transformations/Radians to Degrees
  Throttles : Selector  InputPortWidth=9  Indices=[1,4,7]
  "angles " : Selector  InputPortWidth=9  Indices=[2,3,5,6,8,9]
  (deg) : Outport
  wires:
  (rad)/1 -> Throttles/1, "angles "/1
  Throttles/1 -> Demux1/1
  "angles "/1 -> Radians to Degrees/1
  Mux/1 -> (deg)/1
  Radians to Degrees/1 -> Demux/1
  Demux1/1 -> Mux/1
  Demux/1 -> Mux/2
  Demux/2 -> Mux/3
  Demux1/2 -> Mux/4
  Demux/3 -> Mux/5
  Demux/4 -> Mux/6
  Demux1/3 -> Mux/7
  Demux/5 -> Mux/8
  Demux/6 -> Mux/9

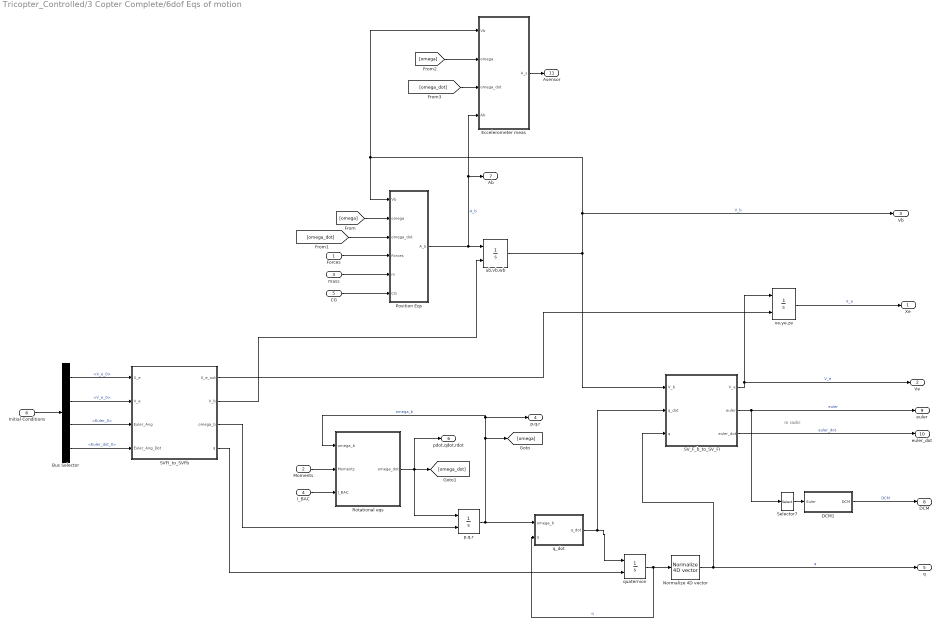
== system Tricopter_Controlled/3 Copter Complete/6dof Eqs of motion ==
  note: In rads!
  Forces : Inport
  Moments : Inport  Port=2
  mass : Inport  Port=3
  I_BAC : Inport  Port=4
  CG : Inport  Port=5
  Initial Conditions : Inport  Port=6
  Bus Selector : BusSelector  OutputSignals=X_e_0,V_e_0,Euler_0,Euler_dot_0
  DCM1 : Subsystem  TreatAsAtomicUnit=on
  Eccelerometer meas : MATLAB Function  TreatAsAtomicUnit=on
      settings: PermitHierarchicalResolution=ParametersOnly
  Normalize 4D vector : XXCopter/Normalize 4D vector
  Position Eqs : MATLAB Function  TreatAsAtomicUnit=on
      settings: PermitHierarchicalResolution=ParametersOnly
  Rotational eqs : MATLAB Function  TreatAsAtomicUnit=on
      settings: PermitHierarchicalResolution=ParametersOnly
  SVFI_to_SVFb : MATLAB Function  TreatAsAtomicUnit=on
      settings: PermitHierarchicalResolution=ParametersOnly
  SV_F_b_to_SV_FI : MATLAB Function  TreatAsAtomicUnit=on
      settings: PermitHierarchicalResolution=ParametersOnly
  Selector7 : Selector  InputPortWidth=3  Indices=[3 2 1]
  "p,q,r " : Integrator  InitialConditionSource=external  InitialCondition=[P_0,Q_0,R_0]
  q_dot : Subsystem  TreatAsAtomicUnit=on
  quaternion : Integrator  InitialConditionSource=external  InitialCondition=[P_0,Q_0,R_0]
  ub,vb,wb : Integrator  InitialConditionSource=external  InitialCondition=[U_0,V_0,W_0]
  xe,ye,ze : Integrator  InitialConditionSource=external  InitialCondition=[NORTH_0,EAST_0,-DOWN_0]
  Xe : Outport
  Ve : Outport  Port=2
  Vb : Outport  Port=3
  p,q,r : Outport  Port=4
  q : Outport  Port=5
  pdot,qdot,rdot : Outport  Port=6
  Ab : Outport  Port=7
  DCM : Outport  Port=8
  euler : Outport  Port=9
  euler_dot : Outport  Port=10
  Asensor : Outport  Port=11
  wires:
  I_BAC/1 -> Rotational eqs/3(I_BAC)
  mass/1 -> Position Eqs/5(m)
  Forces/1 -> Position Eqs/4(Forces)
  xe,ye,ze/1 -> Xe/1  "X_e"
  ub,vb,wb/1 -> Vb/1, Eccelerometer meas/1(Vb), Position Eqs/1(Vb), SV_F_b_to_SV_FI/1(V_b)  "V_b"
  SV_F_b_to_SV_FI/1(V_e) -> Ve/1, xe,ye,ze/1  "V_e"
  [omega] -> Position Eqs/2(omega)
  [omega_dot] -> Position Eqs/3(omega_dot)
  Position Eqs/1(A_b) -> Eccelerometer meas/4(Ab), Ab/1, ub,vb,wb/1  "A_b"
  CG/1 -> Position Eqs/6(CG)
  Initial Conditions/1 -> Bus Selector/1
  Bus Selector/1 -> SVFI_to_SVFb/1(X_e)  "<X_e_0>"
  Bus Selector/2 -> SVFI_to_SVFb/2(V_e)  "<V_e_0>"
  Bus Selector/3 -> SVFI_to_SVFb/3(Euler_Ang)  "<Euler_0>"
  Bus Selector/4 -> SVFI_to_SVFb/4(Euler_Ang_Dot)  "<Euler_dot_0>"
  SVFI_to_SVFb/2(V_b) -> ub,vb,wb/2
  SVFI_to_SVFb/1(X_e_out) -> xe,ye,ze/2
  SVFI_to_SVFb/3(omega_b) -> "p,q,r "/2
  Rotational eqs/1(omega_dot) -> pdot,qdot,rdot/1, [omega_dot], "p,q,r "/1
  "p,q,r "/1 -> q_dot/1(omega_b), [omega], p,q,r/1, Rotational eqs/1(omega_b)  "omega_b"
  q_dot/1(q_dot) -> quaternion/1, SV_F_b_to_SV_FI/2(q_dot)
  SVFI_to_SVFb/4(q) -> quaternion/2
  quaternion/1 -> Normalize 4D vector/1, q_dot/2(q)  "q"
  DCM1/1(DCM) -> DCM/1  "DCM"
  SV_F_b_to_SV_FI/2(euler) -> Selector7/1, euler/1  "euler"
  SV_F_b_to_SV_FI/3(euler_dot) -> euler_dot/1  "euler_dot"
  Moments/1 -> Rotational eqs/2(Moments)
  Normalize 4D vector/1 -> q/1, SV_F_b_to_SV_FI/3(q)  "q"
  [omega] -> Eccelerometer meas/2(omega)
  [omega_dot] -> Eccelerometer meas/3(omega_dot)
  Eccelerometer meas/1(A_s) -> Asensor/1
  Selector7/1 -> DCM1/1(Euler)

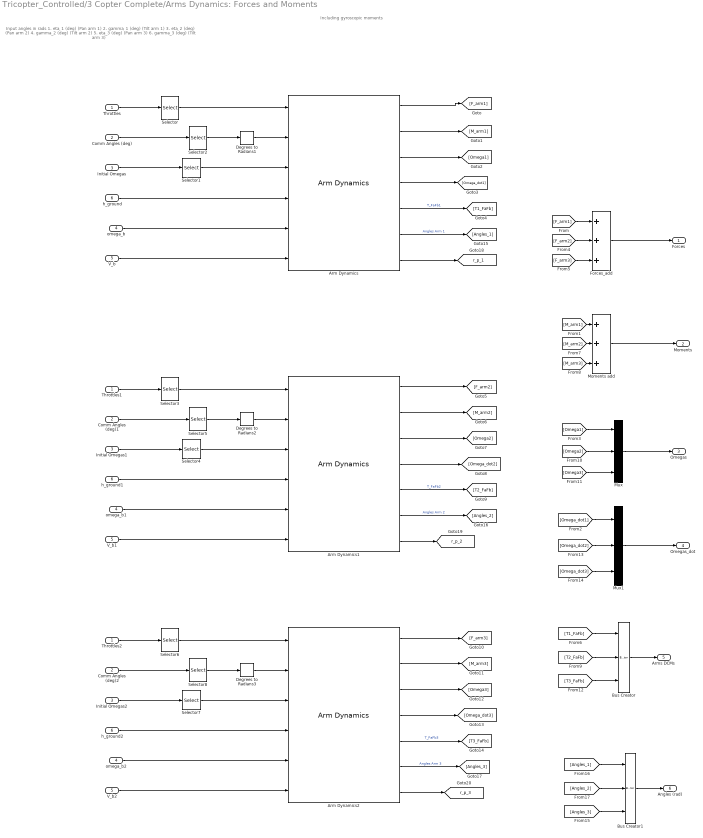
== system Tricopter_Controlled/3 Copter Complete/Arms Dynamics: Forces and Moments ==
  note: Including gyroscopic moments
  note: Input angles in rads
      |
      | 1. eta_1 (deg)  (Pan arm 1)
      | 2. gamma_1 (deg)  (Tilt arm 1)
      |
      | 3. eta_2 (deg)  (Pan arm 2)
      | 4. gamma_2 (deg)  (Tilt arm 2)
      |
      | 5. eta_3 (deg)  (Pan arm  3)
      | 6. gamma_3 (deg)  (Tilt arm 3)
  Throttles : Inport
  Comm Angles (deg) : Inport  Port=2
  Initial Omegas : Inport  Port=3
  omega_b : Inport  Port=4
  V_b : Inport  Port=5
  h_ground : Inport  Port=6
  Arm Dynamics : XXCopter/Arm Dynamics  Rot_sign=Rotation_sign(1)  tau=Tau_motors  arm_hub_pos=l*[1;0;0]  arm_axis=[l_arm;0;0]  arm_num=1  eta_dir=[1;0;0]  gamma_dir=[0;1;0]  J_T=J_T  J_FA=J_FA  h=h  Torq_ini=Initial_Torques(1)  Omega_ini=Initial_Omegas(1)  init_eta=eta_1  init_gamma=0  omega_n=30  xi=1.4  c=0
      link override Arms Kinematics: h_prop=h
  Arm Dynamics1 : XXCopter/Arm Dynamics  Rot_sign=Rotation_sign(2)  tau=Tau_motors  arm_hub_pos=l*[-1/2;sqrt(3)/2;0]  arm_axis=[0;l_arm;0]  arm_num=2  eta_dir=[0;1;0]  gamma_dir=[1;0;0]  J_T=J_T  J_FA=J_FA  h=h  Torq_ini=Initial_Torques(2)  Omega_ini=Initial_Omegas(2)  init_eta=eta_23  init_gamma=0  omega_n=30  xi=1.4  c=0
      link override Arms Kinematics: h_prop=h
  Arm Dynamics2 : XXCopter/Arm Dynamics  Rot_sign=Rotation_sign(3)  tau=Tau_motors  arm_hub_pos=l*[-1/2;-sqrt(3)/2;0]  arm_axis=[0;-l_arm;0]  arm_num=3  eta_dir=[0;1;0]  gamma_dir=[1;0;0]  J_T=J_T  J_FA=J_FA  h=h  Torq_ini=Initial_Torques(3)  Omega_ini=Initial_Omegas(3)  init_eta=-eta_23  init_gamma=0  omega_n=30  xi=1.4  c=0
      link override Arms Kinematics: h_prop=h
  Bus Creator : BusCreator  Inputs=3
  Bus Creator1 : BusCreator  Inputs=3
  Comm Angles (deg)1 : InportShadow  Port=2
  Comm Angles (deg)2 : InportShadow  Port=2
  Degrees to Radians1 : simulink_extras/Transformations/Degrees to Radians
  Degrees to Radians2 : simulink_extras/Transformations/Degrees to Radians
  Degrees to Radians3 : simulink_extras/Transformations/Degrees to Radians
  Forces_add : Sum  Inputs=+++
  Initial Omegas1 : InportShadow  Port=3
  Initial Omegas2 : InportShadow  Port=3
  Moments add : Sum  Inputs=+++
  Mux : Mux  Inputs=3
  Mux1 : Mux  Inputs=3
  Selector : Selector  InputPortWidth=3  Indices=[1]
  Selector1 : Selector  InputPortWidth=3  Indices=[1]
  Selector2 : Selector  InputPortWidth=6  Indices=[1,2]
  Selector3 : Selector  InputPortWidth=3  Indices=2
  Selector4 : Selector  InputPortWidth=3  Indices=2
  Selector5 : Selector  InputPortWidth=6  Indices=[3,4]
  Selector6 : Selector  InputPortWidth=3  Indices=3
  Selector7 : Selector  InputPortWidth=3  Indices=3
  Selector8 : Selector  InputPortWidth=6  Indices=[5,6]
  Throttles1 : InportShadow
  Throttles2 : InportShadow
  V_b1 : InportShadow  Port=5
  V_b2 : InportShadow  Port=5
  h_ground1 : InportShadow  Port=6
  h_ground2 : InportShadow  Port=6
  omega_b1 : InportShadow  Port=4
  omega_b2 : InportShadow  Port=4
  Forces : Outport
  Moments : Outport  Port=2
  Omegas : Outport  Port=3
  Omegas_dot : Outport  Port=4
  Arms DCMs : Outport  Port=5
  Angles (rad) : Outport  Port=6
  tag scope: r_p_1=global, r_p_2=global, r_p_3=global
  wires:
  Selector1/1 -> Arm Dynamics/3
  Throttles/1 -> Selector/1
  Initial Omegas/1 -> Selector1/1
  Selector/1 -> Arm Dynamics/1
  V_b/1 -> Arm Dynamics/6
  Forces_add/1 -> Forces/1
  Moments add/1 -> Moments/1
  Mux/1 -> Omegas/1
  Mux1/1 -> Omegas_dot/1
  h_ground/1 -> Arm Dynamics/4
  Arm Dynamics/1 -> [F_arm1]
  Arm Dynamics/2 -> [M_arm1]
  Arm Dynamics/3 -> [Omega1]
  Arm Dynamics/4 -> [Omega_dot1]
  [F_arm1] -> Forces_add/1
  [M_arm1] -> Moments add/1
  [Omega_dot1] -> Mux1/1
  [Omega1] -> Mux/1
  omega_b/1 -> Arm Dynamics/5
  [F_arm2] -> Forces_add/2
  [F_arm3] -> Forces_add/3
  [Omega2] -> Mux/2
  [Omega3] -> Mux/3
  [Omega_dot2] -> Mux1/2
  [Omega_dot3] -> Mux1/3
  [M_arm3] -> Moments add/3
  [M_arm2] -> Moments add/2
  Degrees to Radians1/1 -> Arm Dynamics/2
  Comm Angles (deg)/1 -> Selector2/1
  Selector2/1 -> Degrees to Radians1/1
  Arm Dynamics/5 -> [T1_FaFb]  "T_FaFb1"
  Bus Creator/1 -> Arms DCMs/1
  [T1_FaFb] -> Bus Creator/1
  Selector4/1 -> Arm Dynamics1/3
  Throttles1/1 -> Selector3/1
  Initial Omegas1/1 -> Selector4/1
  Selector3/1 -> Arm Dynamics1/1
  V_b1/1 -> Arm Dynamics1/6
  h_ground1/1 -> Arm Dynamics1/4
  Arm Dynamics1/1 -> [F_arm2]
  Arm Dynamics1/2 -> [M_arm2]
  Arm Dynamics1/3 -> [Omega2]
  Arm Dynamics1/4 -> [Omega_dot2]
  omega_b1/1 -> Arm Dynamics1/5
  Degrees to Radians2/1 -> Arm Dynamics1/2
  Comm Angles (deg)1/1 -> Selector5/1
  Selector5/1 -> Degrees to Radians2/1
  Arm Dynamics1/5 -> [T2_FaFb]  "T_FaFb2"
  [T2_FaFb] -> Bus Creator/2
  Selector7/1 -> Arm Dynamics2/3
  Throttles2/1 -> Selector6/1
  Initial Omegas2/1 -> Selector7/1
  Selector6/1 -> Arm Dynamics2/1
  V_b2/1 -> Arm Dynamics2/6
  h_ground2/1 -> Arm Dynamics2/4
  Arm Dynamics2/1 -> [F_arm3]
  Arm Dynamics2/2 -> [M_arm3]
  Arm Dynamics2/3 -> [Omega3]
  Arm Dynamics2/4 -> [Omega_dot3]
  omega_b2/1 -> Arm Dynamics2/5
  Degrees to Radians3/1 -> Arm Dynamics2/2
  Comm Angles (deg)2/1 -> Selector8/1
  Selector8/1 -> Degrees to Radians3/1
  Arm Dynamics2/5 -> [T3_FaFb]  "T_FaFb3"
  [T3_FaFb] -> Bus Creator/3
  Bus Creator1/1 -> Angles (rad)/1
  [Angles_1] -> Bus Creator1/1
  [Angles_2] -> Bus Creator1/2
  [Angles_3] -> Bus Creator1/3
  Arm Dynamics/6 -> [Angles_1]  "Angles Arm 1"
  Arm Dynamics1/6 -> [Angles_2]  "Angles Arm 2"
  Arm Dynamics2/6 -> [Angles_3]  "Angles Arm 3"
  Arm Dynamics/7 -> [r_p_1]
  Arm Dynamics1/7 -> [r_p_2]
  Arm Dynamics2/7 -> [r_p_3]

== system Tricopter_Controlled/3 Copter Complete/Contorl Inputs limits ==
  note: limits in degs
  Control inputs : Inport
  Demux : Demux  Outputs=6
  Mux : Mux  Inputs=6
  Saturation : Saturate  UpperLimit=1  LowerLimit=0
  Throttles : Selector  InputPortWidth=9  Indices=[1,4,7]
  "angles " : Selector  InputPortWidth=9  Indices=[2,3,5,6,8,9]
  eta 1 : Saturate  UpperLimit=180  LowerLimit=-180
  eta 2 : Saturate  UpperLimit=180  LowerLimit=-180
  eta 3 : Saturate  UpperLimit=180  LowerLimit=-180
  gamma 2 : Saturate  UpperLimit=90  LowerLimit=-30
  gamma1 : Saturate  UpperLimit=30  LowerLimit=-90
  gamma3 : Saturate  UpperLimit=30  LowerLimit=-90
  Throtles limited : Outport
  Angles limited : Outport  Port=2
  wires:
  Control inputs/1 -> Throttles/1, "angles "/1
  Throttles/1 -> Saturation/1
  "angles "/1 -> Demux/1
  Demux/1 -> eta 1/1
  Demux/2 -> gamma1/1
  Demux/3 -> eta 2/1
  Demux/4 -> gamma 2/1
  Demux/5 -> eta 3/1
  Demux/6 -> gamma3/1
  eta 1/1 -> Mux/1
  gamma1/1 -> Mux/2
  eta 2/1 -> Mux/3
  gamma 2/1 -> Mux/4
  eta 3/1 -> Mux/5
  gamma3/1 -> Mux/6
  Mux/1 -> Angles limited/1
  Saturation/1 -> Throtles limited/1

== system Tricopter_Controlled/3 Copter Complete/Mass Properties ==
  Arms DCMs : Inport
  CG_0 : Inport  Port=2
  m_0 : Inport  Port=3
  m : Inport  Port=4
  m_M : Inport  Port=5
  I_BAC_0 : Inport  Port=6
  Arm Inertia : MATLAB Function  TreatAsAtomicUnit=on
      settings: PermitHierarchicalResolution=ParametersOnly
  Bus Selector : BusSelector  OutputSignals=T_FaFb1,T_FaFb2,T_FaFb3
  CG position : Sum
  Divide : Product  Inputs=*/
  Divide1 : Product  Inputs=**
  Divide2 : Product  Inputs=/*
  Divide3 : Product  Inputs=**
  Motors Pos sum : Sum  Inputs=+++
  Total I_BAC : Sum
  I_BAC : Outport
  CG : Outport  Port=2
  wires:
  Arms DCMs/1 -> Bus Selector/1
  Bus Selector/3 -> Arm Inertia/3(T3_FAFb)  "<T_FaFb3>"
  Bus Selector/2 -> Arm Inertia/2(T2_FAFb)  "<T_FaFb2>"
  Bus Selector/1 -> Arm Inertia/1(T1_FAFb)  "<T_FaFb1>"
  Total I_BAC/1 -> I_BAC/1
  m_0/1 -> Divide/1
  m/1 -> Divide/2, Divide2/1
  CG_0/1 -> Divide1/1
  Divide/1 -> Divide1/2
  m_M/1 -> Divide2/2
  CG position/1 -> CG/1
  Divide1/1 -> CG position/1
  Motors Pos sum/1 -> Divide3/1
  Divide2/1 -> Divide3/2
  Divide3/1 -> CG position/2
  Arm Inertia/3(r2_M) -> Motors Pos sum/2
  Arm Inertia/4(r3_M) -> Motors Pos sum/1
  Arm Inertia/1(I_M) -> Total I_BAC/2
  I_BAC_0/1 -> Total I_BAC/1
  Arm Inertia/2(r1_M) -> Motors Pos sum/3

== system Tricopter_Controlled/Control allocator: NO RECONF/Desired Deflections ==
  Demanded atitude : Inport
  Ground : Ground
  Mux : Mux  Inputs=9
  Trim state : Bias  Bias=[throtle_1,eta_1,0,throtle_23,eta_23,0,throtle_23,-eta_23,0]'
  Unary Minus{,1..5} (6 alike) : UnaryMinus
  phi : Selector  InputPortWidth=3
  theta : Selector  InputPortWidth=3
  Trim deflectins : Outport
  wires:
  Mux/1 -> Trim state/1
  Trim state/1 -> Trim deflectins/1
  Ground/1 -> Mux/7, Mux/4, Mux/1
  Demanded atitude/1 -> phi/1, theta/1
  phi/1 -> Unary Minus5/1, Unary Minus4/1, Unary Minus/1
  Unary Minus/1 -> Mux/2
  Unary Minus1/1 -> Mux/3
  theta/1 -> Unary Minus1/1, Unary Minus2/1, Unary Minus3/1
  Unary Minus2/1 -> Mux/5
  Unary Minus3/1 -> Mux/8
  Unary Minus4/1 -> Mux/6
  Unary Minus5/1 -> Mux/9

== system Tricopter_Controlled/Control allocator: NO RECONF/Hover trim ==
  Ground1 : Ground
  Trim state : Bias  Bias=[throtle_1,eta_1,0,throtle_23,eta_23,0,throtle_23,-eta_23,0]'
  Trim deflectins : Outport
  wires:
  Trim state/1 -> Trim deflectins/1
  Ground1/1 -> Trim state/1

== system Tricopter_Controlled/FlightGear visualization/Flat Earth to LLA ==
  note: Flat Earth to LLA
  Xe : Inport
  altitude0 : Inport  Port=2
  Add : Sum
  Demux2 : Demux  Outputs=2
  Mux : Mux  Inputs=2
  Selector : Selector  InputPortWidth=3  Indices=3
  Unary Minus : UnaryMinus
  deg2rad : Gain  Gain=pi/180  SaturateOnIntegerOverflow=on  OutDataTypeStr=Inherit: Same as input  ParamDataTypeStr=Inherit: Same as input
  ne to lat/long : Subsystem  AncestorBlock=navlibrary/ne to lat//long
  latitude mu : Outport
  longitude l : Outport  Port=2
  altitude h : Outport  Port=3
  wires:
  Demux2/1 -> latitude mu/1  "latitude"
  Demux2/2 -> longitude l/1
  deg2rad/1 -> Demux2/1
  ne to lat/long/1(lat_deg) -> Mux/1
  ne to lat/long/2(long_deg) -> Mux/2
  Mux/1 -> deg2rad/1
  Selector/1 -> Unary Minus/1
  Add/1 -> altitude h/1
  altitude0/1 -> Add/2
  Xe/1 -> ne to lat/long/1(Xe), Selector/1
  Unary Minus/1 -> Add/1

== system Tricopter_Controlled/FlightGear visualization/keep pi//pi ==
  phi theta psi : Inport
  Constant : Constant  Value=180
  Constant2 : Constant  Value=360
  Gain : Gain  Gain=360
  Math Function2 : Math  Operator=rem  SaturateOnIntegerOverflow=on
  Product : Product  Inputs=*/  RndMeth=Zero
  Rounding Function : Rounding  Operator=fix
  Sum2 : Sum  Inputs=|-+
  deg2rad1 : Gain  Gain=pi/180  SaturateOnIntegerOverflow=on  OutDataTypeStr=Inherit: Same as input  ParamDataTypeStr=Inherit: Same as input
  rad2deg : Gain  Gain=180/pi  SaturateOnIntegerOverflow=on  OutDataTypeStr=Inherit: Same as input  ParamDataTypeStr=Inherit: Same as input
  ptp_earth : Outport
  wires:
  phi theta psi/1 -> rad2deg/1
  Constant/1 -> Product/2
  Product/1 -> Rounding Function/1
  Rounding Function/1 -> Gain/1
  Gain/1 -> Sum2/1
  rad2deg/1 -> Math Function2/1
  Constant2/1 -> Math Function2/2
  Math Function2/1 -> Product/1, Sum2/2
  Sum2/1 -> deg2rad1/1
  deg2rad1/1 -> ptp_earth/1

== system Tricopter_Controlled/FlightGear visualization1/Flat Earth to LLA ==
  note: Flat Earth to LLA
  Xe : Inport
  altitude0 : Inport  Port=2
  Angle Conversion : aerolibconvert2/Angle Conversion  IU=deg  OU=rad
  Demux2 : Demux  Outputs=2
  Demux6 : Demux  Outputs=[2 1]
  Display : Display
  Flat Earth to LLA : aerolibtransform2/Flat Earth to LLA  units=Metric (MKS)  ptype=Earth (WGS84)  F=1/298.257223563  R=6378137  LL0=[latitude longitude]  psi=0
  Gain : Gain  Gain=-1
  Mux : Mux  Inputs=2
  longitude l : Outport
  latitude mu : Outport  Port=2
  altitude h : Outport  Port=3
  wires:
  Gain/1 -> Mux/2
  Demux6/2 -> Gain/1
  Demux6/1 -> Mux/1
  Mux/1 -> Flat Earth to LLA/1
  Angle Conversion/1 -> Demux2/1
  Flat Earth to LLA/2 -> altitude h/1, Display/1  "altitude"
  altitude0/1 -> Flat Earth to LLA/2
  Xe/1 -> Demux6/1
  Demux2/2 -> longitude l/1
  Demux2/1 -> latitude mu/1  "latitude"
  Flat Earth to LLA/1 -> Angle Conversion/1

== system Tricopter_Controlled/FlightGear visualization1/phidot thetadot psidot ==
  pqr : Inport
  phi theta psi : Inport  Port=2
  Concatenate1 : Concatenate  NumInputs=3
  Concatenate2 : Concatenate  NumInputs=3
  SinCos : aerolibobsolete/SinCos
  keep angles in range [-pi pi] : Trigonometry  Operator=atan2
  phidot : Fcn  Expr=u[1]+(u[2]*u[4]+u[3]*u[7])*(u[5]/u[8])
  psidot : Fcn  Expr=(u[2]*u[4]+u[3]*u[7])/u[8]
  thetadot : Fcn  Expr=u[2]*u[7]-u[3]*u[4]
  ptp_earth : Outport
  ptp_dot : Outport  Port=2
  wires:
  keep angles in range [-pi pi]/1 -> ptp_earth/1
  Concatenate1/1 -> psidot/1, phidot/1, thetadot/1
  pqr/1 -> Concatenate1/1
  phi theta psi/1 -> SinCos/1
  psidot/1 -> Concatenate2/3
  thetadot/1 -> Concatenate2/2
  phidot/1 -> Concatenate2/1
  Concatenate2/1 -> ptp_dot/1
  SinCos/1 -> keep angles in range [-pi pi]/1, Concatenate1/2
  SinCos/2 -> keep angles in range [-pi pi]/2, Concatenate1/3
